simulink model "Calc"  (R2021a)
settings: Solver=VariableStepAuto  StartTime=0.0  StopTime=10.0  RelTol=1e-3
settings Model: Creator=pc  LastModifiedBy=pc

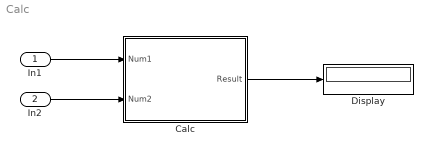
== system Calc ==
  In1 : Inport
  In2 : Inport  Port=2
  Calc : Stateflow chart  TreatAsAtomicUnit=on
  Display : Display
  wires:
  In1/1 -> Calc/1(Num1)
  In2/1 -> Calc/2(Num2)
  Calc/1(Result) -> Display/1

== stateflow chart Calc/Calc ==
  state ?
  state ?
  (default) -> (junction 31) : % Calc Operator
  ? -> ?
  (junction 31) -> (junction 32) [order 1] : [OP == Add]
  (junction 31) -> (junction 35) [order 2]
  (junction 32) -> (junction 33) : {OP==0;}
  (junction 33) -> (junction 34)
  (junction 34) -> (junction 38)
  (junction 35) -> (junction 36) [order 1] : [OP == Sub]
  (junction 35) -> (junction 39) [order 2]
  (junction 36) -> (junction 37) : {OP==1;}
  (junction 37) -> (junction 38)
  (junction 38) -> (junction 42)
  (junction 39) -> (junction 40) [order 1] : [OP == Mul]
  (junction 39) -> (junction 43) [order 2]
  (junction 40) -> (junction 41) : {OP==2;}
  (junction 41) -> (junction 42)
  (junction 42) -> (junction 46)
  (junction 43) -> (junction 44) [order 1] : [OP == Div]
  (junction 43) -> (junction 47) [order 2]
  (junction 44) -> (junction 45) : {OP==3;}
  (junction 45) -> (junction 46)
  (junction 46) -> (junction 48)
  (junction 48) -> (junction 47)
  (junction 47) -> (junction 49)
  data: Num1 input; Num2 input; Result output
